simulink model "pendulum_mdl"  (R2021b)
settings: Solver=FixedStepDiscrete  StartTime=0.0  StopTime=30  FixedStep=0.01  MaxStep=0.25  MinStep=0.01  RelTol=1e-3
values from neighbouring files (symbols this model uses):
  A = [0 1; 0 0]    [pendulum_data.m]
  B = [0;1]    [pendulum_data.m]
  C = C([1,3],:)    [comp_data.m]    (also in pendulum_data.m = [1 1])
  rho = 1    [comp_data.m]    (also in obsint_data.m; obsmod_data.m; outmod_data.m; outmodc_data.m)
undefined symbols (not defined in the file or in its folder): DiscIntNeverNeededParam, Gl, Gn
libraries: simulink x1
settings Model: Creator=w.schwamm  LastModifiedBy=w.schwamm
settings SolverCC: AlgebraicLoopSolver=TrustRegion
settings DataIOCC: SaveOutput=off  SaveTime=off  ReturnWorkspaceOutputs=off  StateSaveName=x  TimeSaveName=t  OutputSaveName=y
settings OptimizationCC: LifeSpan=inf
settings DebuggingCC: SFUnexpectedBacktrackingDiag=warning  SFNoUnconditionalDefaultTransitionDiag=warning  SFMachineParentedDataDiag=warning  ArithmeticOperatorsInVariantConditions=warning
settings SFSimCC: SimUseLocalCustomCode=off  CustomCodeUndefinedFunction=UseInterfaceOnly
settings RTWCC: RTWUseLocalCustomCode=off
settings CodeAppCC: StateflowObjectComments=on
settings GRTTargetCC: TargetLangStandard=C89/C90 (ANSI)
settings ConfigComp: CovMetricSettings=dw  CovSaveCumulativeToWorkspaceVar=on  CovSaveSingleToWorkspaceVar=on  CovExternalEMLEnable=off

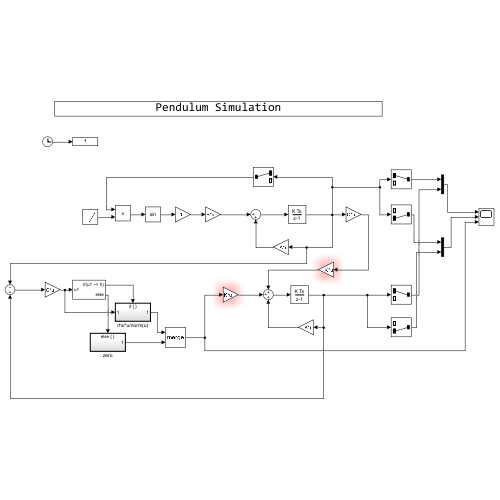
[thumbnail: Simulink's stored preview of the top-level diagram]
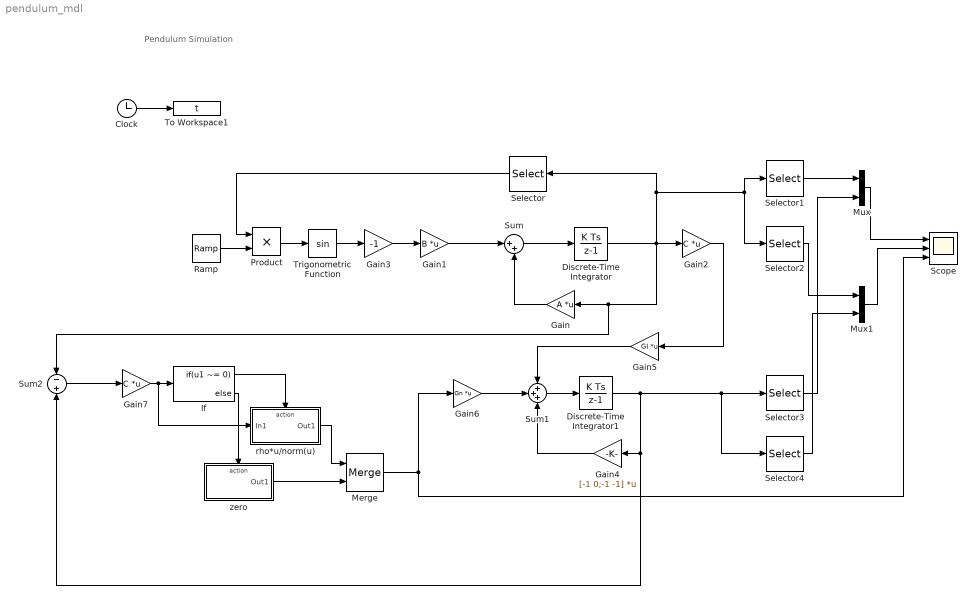
== system pendulum_mdl ==
  note: Pendulum Simulation
  Clock : Clock
  Discrete-Time Integrator : DiscreteIntegrator  InitialCondition=[0.1 0]  SampleTime=-1  ICPrevOutput=DiscIntNeverNeededParam  ICPrevScaledInput=DiscIntNeverNeededParam
  Discrete-Time Integrator1 : DiscreteIntegrator  InitialCondition=[0 0]  SampleTime=-1  ICPrevOutput=DiscIntNeverNeededParam  ICPrevScaledInput=DiscIntNeverNeededParam
  Gain : Gain  Gain=A  Multiplication=Matrix(K*u)
  Gain1 : Gain  Gain=B  Multiplication=Matrix(K*u)
  Gain2 : Gain  Gain=C  Multiplication=Matrix(K*u)
  Gain3 : Gain  Gain=-1
  Gain4 : Gain  Gain=[-1 0;-1 -1]  Multiplication=Matrix(K*u)
  Gain5 : Gain  Gain=Gl  Multiplication=Matrix(K*u)
  Gain6 : Gain  Gain=Gn  Multiplication=Matrix(K*u)
  Gain7 : Gain  Gain=C  Multiplication=Matrix(K*u)
  If : If  IfExpression=u1 ~= 0
  Merge : Merge
  Mux : Mux  Inputs=2
  Mux1 : Mux  Inputs=2
  Product : Product
  Ramp : simulink/Sources/Ramp  slope=0  start=0  InitialOutput=1
  Scope : Scope  NumInputPorts=3
  Selector : Selector  InputPortWidth=2  IndexOptions=Index vector (dialog)  Indices=[1]  OutputSizes=1
  Selector1 : Selector  InputPortWidth=2  IndexOptions=Index vector (dialog)  Indices=[1]  OutputSizes=1
  Selector2 : Selector  InputPortWidth=2  IndexOptions=Index vector (dialog)  Indices=[2]  OutputSizes=1
  Selector3 : Selector  InputPortWidth=2  IndexOptions=Index vector (dialog)  Indices=[1]  OutputSizes=1
  Selector4 : Selector  InputPortWidth=2  IndexOptions=Index vector (dialog)  Indices=[2]  OutputSizes=1
  Sum : Sum  Inputs=|++
  Sum1 : Sum  Inputs=+++
  Sum2 : Sum  Inputs=-+
  To Workspace1 : ToWorkspace  VariableName=t  SaveFormat=Timeseries  SampleTime=-1
      settings: MaxDataPoints=1000000
  Trigonometric Function : Trigonometry
  rho*u/norm(u) : Subsystem  TreatAsAtomicUnit=on
  zero : Subsystem  TreatAsAtomicUnit=on
  wires:
  Clock/1 -> To Workspace1/1
  Gain/1 -> Sum/2
  Sum/1 -> Discrete-Time Integrator/1
  Gain1/1 -> Sum/1
  Selector/1 -> Product/1
  Gain3/1 -> Gain1/1
  Sum1/1 -> Discrete-Time Integrator1/1
  Gain4/1 -> Sum1/3
  Discrete-Time Integrator1/1 -> Selector4/1, Selector3/1, Gain4/1, Sum2/2
  Gain5/1 -> Sum1/1
  Mux/1 -> Scope/1
  Mux1/1 -> Scope/2
  Selector1/1 -> Mux/1
  Selector3/1 -> Mux/2
  Selector2/1 -> Mux1/1
  Selector4/1 -> Mux1/2
  Gain2/1 -> Gain5/1
  Discrete-Time Integrator/1 -> Selector1/1, Selector2/1, Selector/1, Gain2/1, Sum2/1, Gain/1
  Sum2/1 -> Gain7/1
  Gain7/1 -> rho*u/norm(u)/1(In1), If/1
  If/1 -> rho*u/norm(u)/Action
  rho*u/norm(u)/1(Out1) -> Merge/1
  zero/1(Out1) -> Merge/2
  If/2 -> zero/Action
  Gain6/1 -> Sum1/2
  Merge/1 -> Scope/3, Gain6/1
  Trigonometric Function/1 -> Gain3/1
  Product/1 -> Trigonometric Function/1
  Ramp/1 -> Product/2

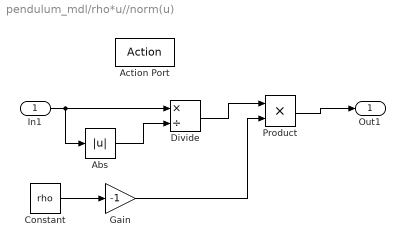
== system pendulum_mdl/rho*u//norm(u) ==
  In1 : Inport
  Action Port : ActionPort  ActionPortLabel=if { }
  Abs : Abs
  Constant : Constant  Value=rho  SampleTime=-1
  Divide : Product  Inputs=*/
  Gain : Gain  Gain=-1
  Product : Product
  Out1 : Outport
  wires:
  Constant/1 -> Gain/1
  In1/1 -> Abs/1, Divide/1
  Abs/1 -> Divide/2
  Divide/1 -> Product/1
  Gain/1 -> Product/2
  Product/1 -> Out1/1

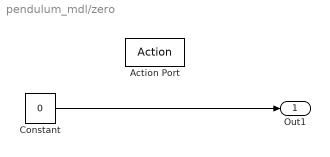
== system pendulum_mdl/zero ==
  Action Port : ActionPort  ActionPortLabel=else { }
  Constant : Constant  Value=0  SampleTime=-1
  Out1 : Outport
  wires:
  Constant/1 -> Out1/1
